simulink model "log_map_tl"  (Simulink 7.5)
settings: Solver=FixedStepDiscrete  StartTime=0.0  StopTime=50.0  FixedStep=0.1  RelTol=1e-3
PreLoadFcn:
  | if exist('tl_preloadfcn','file'), tl_preloadfcn(gcs,101); end
PostLoadFcn:
  | if exist('tl_postloadfcn','file'), tl_postloadfcn(gcs,101); end
InitFcn:
  | if exist('tlds_init','file'), tlds_init(gcs); end
StartFcn:
  | if exist('tlds_start','file'), tlds_start(gcs); end
StopFcn:
  | if exist('tlds_stop','file'), tlds_stop(gcs); end
values from neighbouring files (symbols this model uses):
  alpha = 0.2    [logmap_start.m]
  beta = 0.7    [logmap_start.m]
  lambda = 4.0    (= 4)    [logmap_start.m]
  y1_0 = 0.23421    [logmap_start.m]
  y2_0 = 0.86567    [logmap_start.m]
libraries: tllib x6
PreSaveFcn:
  | if exist('tl_presavefcn','file'), tl_presavefcn(gcs); end
settings Model: DS_PROJECTFILE=log_map_tl.dd  TL_MAIN_DATA={'#advcodeopt',0,'frameopt',{'mexargs',''},'logopt',{'plotinterval',0.1},'date',735991.67651606479}  TL_MODEL_COMMENT=Type in your documentation HERE  TLRevision=101  Creator=alex  LastModifiedBy=alex  BufferReuse=off
settings DataIOCC: LimitDataPoints=off  SaveOutput=off  SaveTime=off
settings OptimizationCC: BlockReduction=off  BooleanDataType=off  OptimizeBlockIOStorage=off  BufferReuse=off  ExpressionFolding=off  LocalBlockOutputs=off  InitFltsAndDblsToZero=on
settings DebuggingCC: SaveWithParameterizedLinksMsg=none  SignalResolutionControl=TryResolveAllWithWarning  SolverPrmCheckMsg=none  MultiTaskDSMMsg=warning  MultiTaskCondExecSysMsg=none
settings HardwareCC: TargetUnknown=on
settings RTWCC: IncludeERTFirstTime=on
settings GRTTargetCC: TargetFcnLib=ansi_tfl_tmw.mat  ModelReferenceCompliant=off  MatFileLogging=off

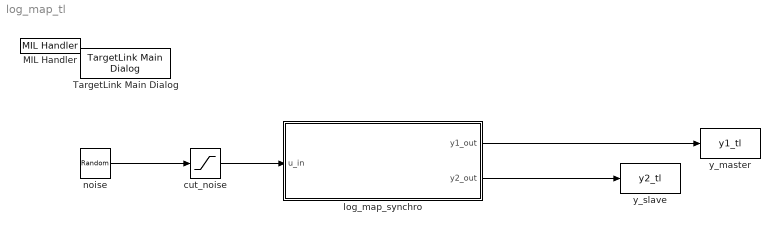
== system log_map_tl ==
  MIL Handler : tllib/MIL Handler  data={'date',735991.67651435186}
  TargetLink Main Dialog : tllib/TargetLink Main Dialog  SystemSampleTime=-1
  cut_noise : Saturate  UpperLimit=1  LowerLimit=0
  log_map_synchro : Subsystem  Tag=TargetLink Simulation Frame
      settings: CopyFcn=if exist('tl_copyfcn','file'), tl_copyfcn(gcbh); end  NameChangeFcn=if exist('tl_framenamechangefcn','file'), tl_framenamechangefcn(gcbh); end
      settings: OpenFcn=|
      | if exist('open_tlsubsystem','file')
      |    open_tlsubsystem(gcbh);
      | else
      |    tlsubsystem = ...
      |       find_system(gcb, ...
      |       'LookUnderMasks','on', ...
      |       'FollowLinks','on', ...
      |       'Tag','MIL Subsystem');
      |    open_system(tlsubsystem);
      | end
      mask Type: TL_SimFrame
      mask Display: disp('TargetLink\nModel-\nin-the-loop\nmode')
  noise : RandomNumber  Mean=0.5  SampleTime=0
  y_master : ToWorkspace  VariableName=y1_tl  SampleTime=-1  SaveFormat=Array
  y_slave : ToWorkspace  VariableName=y2_tl  SampleTime=-1  SaveFormat=Array
  wires:
  noise/1 -> cut_noise/1
  log_map_synchro/1(y1_out) -> y_master/1
  cut_noise/1 -> log_map_synchro/1(u_in)
  log_map_synchro/2(y2_out) -> y_slave/1

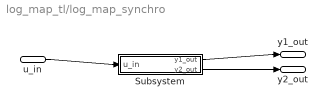
== system log_map_tl/log_map_synchro ==
  u_in : Inport  SampleTime=0.1  OutDataType=sfix(16)  OutScaling=2^0
  Subsystem : Subsystem  Tag=struct('sfcnName','log_map_synchro_sf','subFunction','','srcSubsystem','')
      settings: OpenFcn=warndlg(get_param(gcb,'MaskHelp'),'Serious Warning');
      mask Type: TL_Enable
      mask Help: This subsystem keeps the TargetLink subsystem (subsystem with TargetLink blocks for production code generation), and is needed for the TargetLink simulation frame to work properly. DO NOT DELETE OR MODIFY IT!
  y1_out : Outport  OutDataType=sfix(16)  OutScaling=2^0
  y2_out : Outport  Port=2  OutDataType=sfix(16)  OutScaling=2^0
  wires:
  u_in/1 -> Subsystem/1(u_in)
  Subsystem/1(y1_out) -> y1_out/1
  Subsystem/2(y2_out) -> y2_out/1

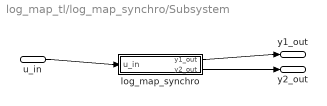
== system log_map_tl/log_map_synchro/Subsystem ==
  u_in : Inport  SampleTime=0.1  OutDataType=sfix(16)  OutScaling=2^0
  log_map_synchro : Subsystem  Tag=MIL Subsystem  Description=b
      settings: CopyFcn=if exist('tl_copyfcn','file'), tl_copyfcn(gcbh); end  NameChangeFcn=if exist('tl_namechangefcn','file'), tl_namechangefcn(gcbh); end  DestroyFcn=if exist('update_tl_main_dlg','file'), update_tl_main_dlg('TL_subs_display'); end
  y1_out : Outport  OutDataType=sfix(16)  OutScaling=2^0
  y2_out : Outport  Port=2  OutDataType=sfix(16)  OutScaling=2^0
  wires:
  u_in/1 -> log_map_synchro/1(u_in)
  log_map_synchro/1(y1_out) -> y1_out/1
  log_map_synchro/2(y2_out) -> y2_out/1

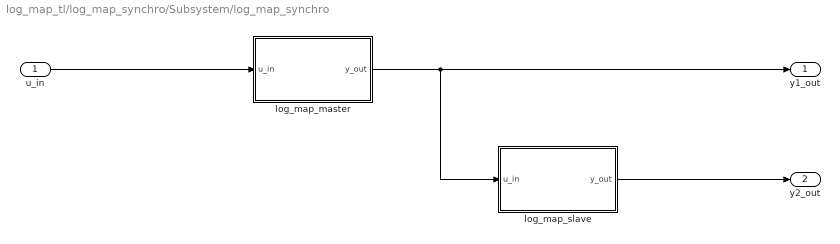
== system log_map_tl/log_map_synchro/Subsystem/log_map_synchro ==
  u_in : Inport  Description=|  PortDimensions=1  SampleTime=0.1  OutDataType=sfix(16)  OutScaling=2^0  mask(TL_Inport){data={'logdata',{'plotchannels',[]},'output',{'max',1,'min',0,'type','UInt16','lsb',2^-15},'date',735991.67651483801}}
      | InPort block of dSPACE TargetLink.
      | 
      | Input signal is read from an external variable and scaled:
      | 
      |         y = lsb * u + offset
      settings: DeleteFcn=if exist('delete_tlblock','file')==2,delete_tlblock(gcbh);end  OpenFcn=if exist('tl_open_blockdlg','file')==2,tl_open_blockdlg(gcbh);else,open_system(gcbh,'parameter');end
      settings: CopyFcn=|
      | if exist('tl_reset_reviewflag','file')==2
      |     tl_reset_reviewflag(gcbh);
      | end
      | if exist('tl_check_ports','file')
      |     tl_check_ports(gcbh);
      | end
      settings: NameChangeFcn=|
      | if exist('rename_tlblock','file')==2,rename_tlblock(gcbh);end
      | if exist('tl_check_ports','file'), tl_check_ports(gcbh); end
      mask Help: eval(['if exist(''tl_online_help'',''file'') == 2, tl_online_help(''Topic'',''TL_Inport''),else, web([''jar:file:///'',matlabroot,''/help/toolbox/simulink/help.jar!/slref/' lower(get_param(gcbh,'Blocktype')) '.html''], ''-helpbrowser''),end'])
      mask Display: plot([0.2 0.35 NaN 0.65 0.8],[0 1 NaN 0 1]);
  log_map_master : Subsystem  TreatAsAtomicUnit=on
  log_map_slave : Subsystem  TreatAsAtomicUnit=on
  y1_out : Outport  Description=|  PortDimensions=1  OutDataType=sfix(16)  OutScaling=2^0  mask(TL_Outport){data={'logdata',{'plotchannels',[]},'output',{'max',1,'min',0,'type','UInt16','lsb',2^-15},'date',735991.67650769674}}
      | OutPort block of dSPACE TargetLink.
      | 
      | Input signal is scaled:
      | 
      |         y = lsb * u + offset
      settings: DeleteFcn=if exist('delete_tlblock','file')==2,delete_tlblock(gcbh);end  OpenFcn=if exist('tl_open_blockdlg','file')==2,tl_open_blockdlg(gcbh);else,open_system(gcbh,'parameter');end
      settings: CopyFcn=|
      | if exist('tl_reset_reviewflag','file')==2
      |     tl_reset_reviewflag(gcbh);
      | end
      | if exist('tl_check_ports','file')
      |     tl_check_ports(gcbh);
      | end
      settings: NameChangeFcn=|
      | if exist('rename_tlblock','file')==2,rename_tlblock(gcbh);end
      | if exist('tl_check_ports','file'), tl_check_ports(gcbh); end
      mask Help: eval(['if exist(''tl_online_help'',''file'') == 2, tl_online_help(''Topic'',''TL_Outport''),else, web([''jar:file:///'',matlabroot,''/help/toolbox/simulink/help.jar!/slref/' lower(get_param(gcbh,'Blocktype')) '.html''], ''-helpbrowser''),end'])
      mask Display: plot([0.2 0.35 NaN 0.65 0.8],[0 1 NaN 0 1]);
  y2_out : Outport  Description=|  Port=2  PortDimensions=1  OutDataType=sfix(16)  OutScaling=2^0  mask(TL_Outport){data={'logdata',{'plotchannels',[]},'output',{'max',1,'min',0,'type','UInt16','lsb',2^-15},'date',735991.67650722223}}
      | OutPort block of dSPACE TargetLink.
      | 
      | Input signal is scaled:
      | 
      |         y = lsb * u + offset
      settings: DeleteFcn=if exist('delete_tlblock','file')==2,delete_tlblock(gcbh);end  OpenFcn=if exist('tl_open_blockdlg','file')==2,tl_open_blockdlg(gcbh);else,open_system(gcbh,'parameter');end
      settings: CopyFcn=|
      | if exist('tl_reset_reviewflag','file')==2
      |     tl_reset_reviewflag(gcbh);
      | end
      | if exist('tl_check_ports','file')
      |     tl_check_ports(gcbh);
      | end
      settings: NameChangeFcn=|
      | if exist('rename_tlblock','file')==2,rename_tlblock(gcbh);end
      | if exist('tl_check_ports','file'), tl_check_ports(gcbh); end
      mask Help: eval(['if exist(''tl_online_help'',''file'') == 2, tl_online_help(''Topic'',''TL_Outport''),else, web([''jar:file:///'',matlabroot,''/help/toolbox/simulink/help.jar!/slref/' lower(get_param(gcbh,'Blocktype')) '.html''], ''-helpbrowser''),end'])
      mask Display: plot([0.2 0.35 NaN 0.65 0.8],[0 1 NaN 0 1]);
  wires:
  log_map_master/1(y_out) -> log_map_slave/1(u_in), y1_out/1
  u_in/1 -> log_map_master/1(u_in)
  log_map_slave/1(y_out) -> y2_out/1

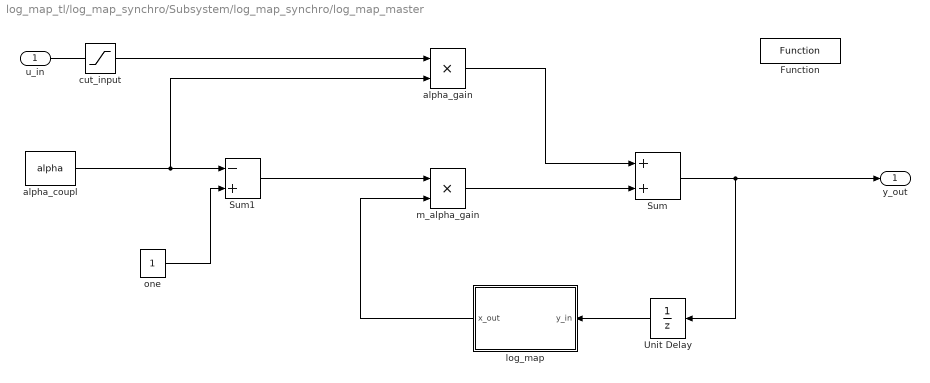
== system log_map_tl/log_map_synchro/Subsystem/log_map_synchro/log_map_master ==
  u_in : Inport  OutDataType=sfix(16)  OutScaling=2^0
  Function : tllib/Function  Description=|  SystemSampleTime=-1  data={'date',735991.6765065972}
      | Function block of dSPACE TargetLink.
      | 
      | Copy this block into a subsystem if you want separate code to be generated for it.
  Sum : Sum  Description=|  OutDataType=sfix(16)  OutScaling=2^-10  mask(TL_Sum){data={'logdata',{'plotchannels',[]},'output',{'max',1,'min',0,'type','UInt16','lsb',2^-15},'date',735991.67651423614}}
      | Sum block of dSPACE TargetLink.
      | 
      | Output signal is equal to the sum of the input signals.
      | The list of signs is specified according to conventions for Simulink Sum blocks.
      settings: CopyFcn=set_param(gcb,'ReferenceBlock',''); set_param(gcb,'Tag','COPIED_DURING_UPGRADE');set_param(gcb,'CopyFcn','');  DeleteFcn=if exist('delete_tlblock','file')==2,delete_tlblock(gcbh);end  NameChangeFcn=if exist('rename_tlblock','file')==2,rename_tlblock(gcbh);end  OpenFcn=if exist('tl_open_blockdlg','file')==2,tl_open_blockdlg(gcbh);else,open_system(gcbh,'parameter');end
      mask Help: eval(['if exist(''tl_online_help'',''file'') == 2, tl_online_help(''Topic'',''TL_Sum''),else, web([''jar:file:///'',matlabroot,''/help/toolbox/simulink/help.jar!/slref/' lower(get_param(gcbh,'Blocktype')) '.html''], ''-helpbrowser''),end'])
      mask Display: plot([-0.05, 1.05, NaN, -0.05, 1.05],[.01, .01, NaN, .99, .99])
  Sum1 : Sum  Description=|  Inputs=-+  OutDataType=sfix(16)  OutScaling=2^-10  mask(TL_Sum){data={'logdata',{'plotchannels',[]},'output',{'max',1,'type','UInt16','lsb',2^-15},'date',735991.67651399306}}
      | Sum block of dSPACE TargetLink.
      | 
      | Output signal is equal to the sum of the input signals.
      | The list of signs is specified according to conventions for Simulink Sum blocks.
      settings: CopyFcn=set_param(gcb,'ReferenceBlock',''); set_param(gcb,'Tag','COPIED_DURING_UPGRADE');set_param(gcb,'CopyFcn','');  DeleteFcn=if exist('delete_tlblock','file')==2,delete_tlblock(gcbh);end  NameChangeFcn=if exist('rename_tlblock','file')==2,rename_tlblock(gcbh);end  OpenFcn=if exist('tl_open_blockdlg','file')==2,tl_open_blockdlg(gcbh);else,open_system(gcbh,'parameter');end
      mask Help: eval(['if exist(''tl_online_help'',''file'') == 2, tl_online_help(''Topic'',''TL_Sum''),else, web([''jar:file:///'',matlabroot,''/help/toolbox/simulink/help.jar!/slref/' lower(get_param(gcbh,'Blocktype')) '.html''], ''-helpbrowser''),end'])
      mask Display: plot([-0.05, 1.05, NaN, -0.05, 1.05],[.01, .01, NaN, .99, .99])
  Unit Delay : UnitDelay  Description=|  X0=y1_0  SampleTime=-1  mask(TL_UnitDelay){data={'logdata',{'plotchannels',[]},'output',{'max',1,'min',0,'type','UInt16','lsb',2^-15},'state',{'max',1,'min',0,'type','UInt16','lsb',2^-15},'date',735991.67651372682}}
      | Unit Delay block of dSPACE TargetLink.
      | 
      | Output signal is equal to the input signal of the last sample step:
      | 
      |         y(k) = u(k-1).
      | 
      | In the 1st sampling step, the output signal is initialized with 'initial condition':
      | 
      |         y(0) = initial condition
      settings: CopyFcn=set_param(gcb,'ReferenceBlock',''); set_param(gcb,'Tag','COPIED_DURING_UPGRADE');set_param(gcb,'CopyFcn','');  DeleteFcn=if exist('delete_tlblock','file')==2,delete_tlblock(gcbh);end  NameChangeFcn=if exist('rename_tlblock','file')==2,rename_tlblock(gcbh);end  OpenFcn=if exist('tl_open_blockdlg','file')==2,tl_open_blockdlg(gcbh);else,open_system(gcbh,'parameter');end
      mask Help: eval(['if exist(''tl_online_help'',''file'') == 2, tl_online_help(''Topic'',''TL_UnitDelay''),else, web([''jar:file:///'',matlabroot,''/help/toolbox/simulink/help.jar!/slref/' lower(get_param(gcbh,'Blocktype')) '.html''], ''-helpbrowser''),end'])
      mask Display: plot([-0.05, 1.05, NaN, -0.05, 1.05],[.01, .01, NaN, .99, .99])
  alpha_coupl : Constant  Description=|  Value=alpha  OutDataType=sfix(16)  OutScaling=2^0  mask(TL_Constant){data={'output',{'max',1,'min',0,'class','CAL','type','UInt16','lsb',2^-15},'date',735991.67651340272}}
      | Constant block of dSPACE TargetLink.
      | 
      | Output signal keeps the given constant value.
      settings: CopyFcn=set_param(gcb,'ReferenceBlock',''); set_param(gcb,'Tag','COPIED_DURING_UPGRADE');set_param(gcb,'CopyFcn','');  DeleteFcn=if exist('delete_tlblock','file')==2,delete_tlblock(gcbh);end  NameChangeFcn=if exist('rename_tlblock','file')==2,rename_tlblock(gcbh);end  OpenFcn=if exist('tl_open_blockdlg','file')==2,tl_open_blockdlg(gcbh);else,open_system(gcbh,'parameter');end
      mask Help: eval(['if exist(''tl_online_help'',''file'') == 2, tl_online_help(''Topic'',''TL_Constant''),else, web([''jar:file:///'',matlabroot,''/help/toolbox/simulink/help.jar!/slref/' lower(get_param(gcbh,'Blocktype')) '.html''], ''-helpbrowser''),end'])
      mask Display: plot([-0.05, 1.05, NaN, -0.05, 1.05],[.01, .01, NaN, .99, .99])
  alpha_gain : Product  Description=|  Inputs=**  OutDataType=sfix(16)  OutScaling=2^0  RndMeth=Zero  mask(TL_Product){data={'logdata',{'plotchannels',[]},'output',{'max',1,'min',0,'type','UInt16','lsb',2^-15},'date',735991.67651315976}}
      | Product block of dSPACE TargetLink.
      | 
      | Output signal is equal to the product of the input signals. The input ports are specified according to conventions for Simulink Product blocks.
      settings: CopyFcn=set_param(gcb,'ReferenceBlock',''); set_param(gcb,'Tag','COPIED_DURING_UPGRADE');set_param(gcb,'CopyFcn','');  DeleteFcn=if exist('delete_tlblock','file')==2,delete_tlblock(gcbh);end  NameChangeFcn=if exist('rename_tlblock','file')==2,rename_tlblock(gcbh);end  OpenFcn=if exist('tl_open_blockdlg','file')==2,tl_open_blockdlg(gcbh);else,open_system(gcbh,'parameter');end
      mask Help: eval(['if exist(''tl_online_help'',''file'') == 2, tl_online_help(''Topic'',''TL_Product''),else, web([''jar:file:///'',matlabroot,''/help/toolbox/simulink/help.jar!/slref/' lower(get_param(gcbh,'Blocktype')) '.html''], ''-helpbrowser''),end'])
      mask Display: plot([-0.05, 1.05, NaN, -0.05, 1.05],[.01, .01, NaN, .99, .99])
  cut_input : Saturate  Description=|  UpperLimit=1  LowerLimit=0  OutDataType=sfix(16)  OutScaling=2^0  mask(TL_Saturate){data={'logdata',{'plotchannels',[]},'output',{'max',1,'min',0,'type','UInt16','lsb',2^-15},'lowerlimit',{'class','GLOBAL','type','UInt16','lsb',2^-15},'upperlimit',{'class','GLOBAL','type','UInt16','lsb',2^-15},'date',735991.676512882}}
      | Saturation block of dSPACE TargetLink.
      | 
      | The Saturation block saturates its input to the given upper and lower limit.
      settings: CopyFcn=set_param(gcb,'ReferenceBlock',''); set_param(gcb,'Tag','COPIED_DURING_UPGRADE');set_param(gcb,'CopyFcn','');  DeleteFcn=if exist('delete_tlblock','file')==2,delete_tlblock(gcbh);end  NameChangeFcn=if exist('rename_tlblock','file')==2,rename_tlblock(gcbh);end  OpenFcn=if exist('tl_open_blockdlg','file')==2,tl_open_blockdlg(gcbh);else,open_system(gcbh,'parameter');end
      mask Help: eval(['if exist(''tl_online_help'',''file'') == 2, tl_online_help(''Topic'',''TL_Saturate''),else, web([''jar:file:///'',matlabroot,''/help/toolbox/simulink/help.jar!/slref/' lower(get_param(gcbh,'Blocktype')) '.html''], ''-helpbrowser''),end'])
      mask Display: plot([-0.05, 1.05, NaN, -0.05, 1.05],[.01, .01, NaN, .99, .99])
  log_map : Subsystem  TreatAsAtomicUnit=on
  m_alpha_gain : Product  Description=|  Inputs=**  OutDataType=sfix(16)  OutScaling=2^0  RndMeth=Zero  mask(TL_Product){data={'logdata',{'plotchannels',[]},'output',{'max',1,'min',0,'type','UInt16','lsb',2^-15},'date',735991.67651142366}}
      | Product block of dSPACE TargetLink.
      | 
      | Output signal is equal to the product of the input signals. The input ports are specified according to conventions for Simulink Product blocks.
      settings: CopyFcn=set_param(gcb,'ReferenceBlock',''); set_param(gcb,'Tag','COPIED_DURING_UPGRADE');set_param(gcb,'CopyFcn','');  DeleteFcn=if exist('delete_tlblock','file')==2,delete_tlblock(gcbh);end  NameChangeFcn=if exist('rename_tlblock','file')==2,rename_tlblock(gcbh);end  OpenFcn=if exist('tl_open_blockdlg','file')==2,tl_open_blockdlg(gcbh);else,open_system(gcbh,'parameter');end
      mask Help: eval(['if exist(''tl_online_help'',''file'') == 2, tl_online_help(''Topic'',''TL_Product''),else, web([''jar:file:///'',matlabroot,''/help/toolbox/simulink/help.jar!/slref/' lower(get_param(gcbh,'Blocktype')) '.html''], ''-helpbrowser''),end'])
      mask Display: plot([-0.05, 1.05, NaN, -0.05, 1.05],[.01, .01, NaN, .99, .99])
  one : Constant  Description=|  OutDataType=sfix(16)  OutScaling=2^0  mask(TL_Constant){data={'output',{'class','CONST','type','UInt16','lsb',2^-15,'tolerance',0.001},'date',735991.67651119211}}
      | Constant block of dSPACE TargetLink.
      | 
      | Output signal keeps the given constant value.
      settings: CopyFcn=set_param(gcb,'ReferenceBlock',''); set_param(gcb,'Tag','COPIED_DURING_UPGRADE');set_param(gcb,'CopyFcn','');  DeleteFcn=if exist('delete_tlblock','file')==2,delete_tlblock(gcbh);end  NameChangeFcn=if exist('rename_tlblock','file')==2,rename_tlblock(gcbh);end  OpenFcn=if exist('tl_open_blockdlg','file')==2,tl_open_blockdlg(gcbh);else,open_system(gcbh,'parameter');end
      mask Help: eval(['if exist(''tl_online_help'',''file'') == 2, tl_online_help(''Topic'',''TL_Constant''),else, web([''jar:file:///'',matlabroot,''/help/toolbox/simulink/help.jar!/slref/' lower(get_param(gcbh,'Blocktype')) '.html''], ''-helpbrowser''),end'])
      mask Display: plot([-0.05, 1.05, NaN, -0.05, 1.05],[.01, .01, NaN, .99, .99])
  y_out : Outport  OutDataType=sfix(16)  OutScaling=2^0
  wires:
  cut_input/1 -> alpha_gain/1
  m_alpha_gain/1 -> Sum/2
  alpha_gain/1 -> Sum/1
  log_map/1(x_out) -> m_alpha_gain/2
  Sum/1 -> y_out/1, Unit Delay/1
  u_in/1 -> cut_input/1
  Unit Delay/1 -> log_map/1(y_in)
  one/1 -> Sum1/2
  Sum1/1 -> m_alpha_gain/1
  alpha_coupl/1 -> Sum1/1, alpha_gain/2

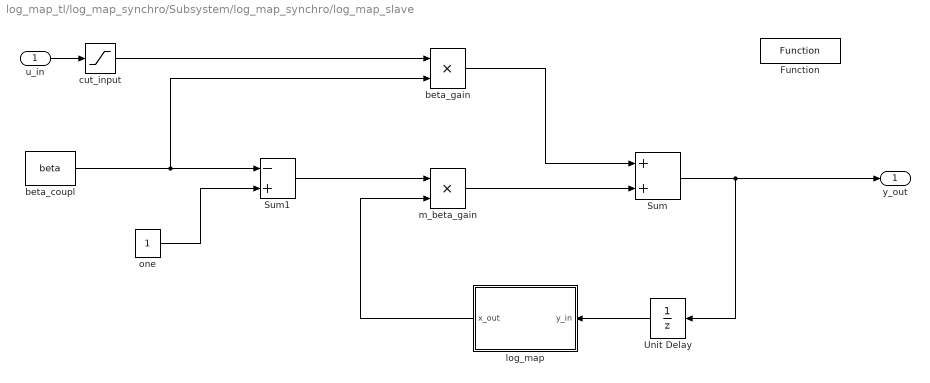
== system log_map_tl/log_map_synchro/Subsystem/log_map_synchro/log_map_slave ==
  u_in : Inport  OutDataType=sfix(16)  OutScaling=2^0
  Function : tllib/Function  Description=|  SystemSampleTime=-1  data={'date',735991.67650611117}
      | Function block of dSPACE TargetLink.
      | 
      | Copy this block into a subsystem if you want separate code to be generated for it.
  Sum : Sum  Description=|  OutDataType=sfix(16)  OutScaling=2^-10  mask(TL_Sum){data={'logdata',{'plotchannels',[]},'output',{'max',1,'min',0,'type','UInt16','lsb',2^-15},'date',735991.67651094904}}
      | Sum block of dSPACE TargetLink.
      | 
      | Output signal is equal to the sum of the input signals.
      | The list of signs is specified according to conventions for Simulink Sum blocks.
      settings: CopyFcn=set_param(gcb,'ReferenceBlock',''); set_param(gcb,'Tag','COPIED_DURING_UPGRADE');set_param(gcb,'CopyFcn','');  DeleteFcn=if exist('delete_tlblock','file')==2,delete_tlblock(gcbh);end  NameChangeFcn=if exist('rename_tlblock','file')==2,rename_tlblock(gcbh);end  OpenFcn=if exist('tl_open_blockdlg','file')==2,tl_open_blockdlg(gcbh);else,open_system(gcbh,'parameter');end
      mask Help: eval(['if exist(''tl_online_help'',''file'') == 2, tl_online_help(''Topic'',''TL_Sum''),else, web([''jar:file:///'',matlabroot,''/help/toolbox/simulink/help.jar!/slref/' lower(get_param(gcbh,'Blocktype')) '.html''], ''-helpbrowser''),end'])
      mask Display: plot([-0.05, 1.05, NaN, -0.05, 1.05],[.01, .01, NaN, .99, .99])
  Sum1 : Sum  Description=|  Inputs=-+  OutDataType=sfix(16)  OutScaling=2^-10  mask(TL_Sum){data={'logdata',{'plotchannels',[]},'output',{'max',1,'type','UInt16','lsb',2^-15},'date',735991.67651068291}}
      | Sum block of dSPACE TargetLink.
      | 
      | Output signal is equal to the sum of the input signals.
      | The list of signs is specified according to conventions for Simulink Sum blocks.
      settings: CopyFcn=set_param(gcb,'ReferenceBlock',''); set_param(gcb,'Tag','COPIED_DURING_UPGRADE');set_param(gcb,'CopyFcn','');  DeleteFcn=if exist('delete_tlblock','file')==2,delete_tlblock(gcbh);end  NameChangeFcn=if exist('rename_tlblock','file')==2,rename_tlblock(gcbh);end  OpenFcn=if exist('tl_open_blockdlg','file')==2,tl_open_blockdlg(gcbh);else,open_system(gcbh,'parameter');end
      mask Help: eval(['if exist(''tl_online_help'',''file'') == 2, tl_online_help(''Topic'',''TL_Sum''),else, web([''jar:file:///'',matlabroot,''/help/toolbox/simulink/help.jar!/slref/' lower(get_param(gcbh,'Blocktype')) '.html''], ''-helpbrowser''),end'])
      mask Display: plot([-0.05, 1.05, NaN, -0.05, 1.05],[.01, .01, NaN, .99, .99])
  Unit Delay : UnitDelay  Description=|  X0=y2_0  SampleTime=-1  mask(TL_UnitDelay){data={'logdata',{'plotchannels',[]},'output',{'max',1,'min',0,'type','UInt16','lsb',2^-15},'state',{'max',1,'min',0,'type','UInt16','lsb',2^-15},'date',735991.67651043984}}
      | Unit Delay block of dSPACE TargetLink.
      | 
      | Output signal is equal to the input signal of the last sample step:
      | 
      |         y(k) = u(k-1).
      | 
      | In the 1st sampling step, the output signal is initialized with 'initial condition':
      | 
      |         y(0) = initial condition
      settings: CopyFcn=set_param(gcb,'ReferenceBlock',''); set_param(gcb,'Tag','COPIED_DURING_UPGRADE');set_param(gcb,'CopyFcn','');  DeleteFcn=if exist('delete_tlblock','file')==2,delete_tlblock(gcbh);end  NameChangeFcn=if exist('rename_tlblock','file')==2,rename_tlblock(gcbh);end  OpenFcn=if exist('tl_open_blockdlg','file')==2,tl_open_blockdlg(gcbh);else,open_system(gcbh,'parameter');end
      mask Help: eval(['if exist(''tl_online_help'',''file'') == 2, tl_online_help(''Topic'',''TL_UnitDelay''),else, web([''jar:file:///'',matlabroot,''/help/toolbox/simulink/help.jar!/slref/' lower(get_param(gcbh,'Blocktype')) '.html''], ''-helpbrowser''),end'])
      mask Display: plot([-0.05, 1.05, NaN, -0.05, 1.05],[.01, .01, NaN, .99, .99])
  beta_coupl : Constant  Description=|  Value=beta  OutDataType=sfix(16)  OutScaling=2^0  mask(TL_Constant){data={'output',{'max',1,'min',0,'class','CAL','type','UInt16','lsb',2^-15},'date',735991.67651011574}}
      | Constant block of dSPACE TargetLink.
      | 
      | Output signal keeps the given constant value.
      settings: CopyFcn=set_param(gcb,'ReferenceBlock',''); set_param(gcb,'Tag','COPIED_DURING_UPGRADE');set_param(gcb,'CopyFcn','');  DeleteFcn=if exist('delete_tlblock','file')==2,delete_tlblock(gcbh);end  NameChangeFcn=if exist('rename_tlblock','file')==2,rename_tlblock(gcbh);end  OpenFcn=if exist('tl_open_blockdlg','file')==2,tl_open_blockdlg(gcbh);else,open_system(gcbh,'parameter');end
      mask Help: eval(['if exist(''tl_online_help'',''file'') == 2, tl_online_help(''Topic'',''TL_Constant''),else, web([''jar:file:///'',matlabroot,''/help/toolbox/simulink/help.jar!/slref/' lower(get_param(gcbh,'Blocktype')) '.html''], ''-helpbrowser''),end'])
      mask Display: plot([-0.05, 1.05, NaN, -0.05, 1.05],[.01, .01, NaN, .99, .99])
  beta_gain : Product  Description=|  Inputs=**  OutDataType=sfix(16)  OutScaling=2^0  RndMeth=Zero  mask(TL_Product){data={'logdata',{'plotchannels',[]},'output',{'max',1,'min',0,'type','UInt16','lsb',2^-15},'date',735991.67650987266}}
      | Product block of dSPACE TargetLink.
      | 
      | Output signal is equal to the product of the input signals. The input ports are specified according to conventions for Simulink Product blocks.
      settings: CopyFcn=set_param(gcb,'ReferenceBlock',''); set_param(gcb,'Tag','COPIED_DURING_UPGRADE');set_param(gcb,'CopyFcn','');  DeleteFcn=if exist('delete_tlblock','file')==2,delete_tlblock(gcbh);end  NameChangeFcn=if exist('rename_tlblock','file')==2,rename_tlblock(gcbh);end  OpenFcn=if exist('tl_open_blockdlg','file')==2,tl_open_blockdlg(gcbh);else,open_system(gcbh,'parameter');end
      mask Help: eval(['if exist(''tl_online_help'',''file'') == 2, tl_online_help(''Topic'',''TL_Product''),else, web([''jar:file:///'',matlabroot,''/help/toolbox/simulink/help.jar!/slref/' lower(get_param(gcbh,'Blocktype')) '.html''], ''-helpbrowser''),end'])
      mask Display: plot([-0.05, 1.05, NaN, -0.05, 1.05],[.01, .01, NaN, .99, .99])
  cut_input : Saturate  Description=|  UpperLimit=1  LowerLimit=0  OutDataType=sfix(16)  OutScaling=2^0  mask(TL_Saturate){data={'logdata',{'plotchannels',[]},'output',{'max',1,'min',0,'type','UInt16','lsb',2^-15},'lowerlimit',{'class','GLOBAL','type','UInt16','lsb',2^-15},'upperlimit',{'class','GLOBAL','type','UInt16','lsb',2^-15},'date',735991.67650961806}}
      | Saturation block of dSPACE TargetLink.
      | 
      | The Saturation block saturates its input to the given upper and lower limit.
      settings: CopyFcn=set_param(gcb,'ReferenceBlock',''); set_param(gcb,'Tag','COPIED_DURING_UPGRADE');set_param(gcb,'CopyFcn','');  DeleteFcn=if exist('delete_tlblock','file')==2,delete_tlblock(gcbh);end  NameChangeFcn=if exist('rename_tlblock','file')==2,rename_tlblock(gcbh);end  OpenFcn=if exist('tl_open_blockdlg','file')==2,tl_open_blockdlg(gcbh);else,open_system(gcbh,'parameter');end
      mask Help: eval(['if exist(''tl_online_help'',''file'') == 2, tl_online_help(''Topic'',''TL_Saturate''),else, web([''jar:file:///'',matlabroot,''/help/toolbox/simulink/help.jar!/slref/' lower(get_param(gcbh,'Blocktype')) '.html''], ''-helpbrowser''),end'])
      mask Display: plot([-0.05, 1.05, NaN, -0.05, 1.05],[.01, .01, NaN, .99, .99])
  log_map : Subsystem  TreatAsAtomicUnit=on
  m_beta_gain : Product  Description=|  Inputs=**  OutDataType=sfix(16)  OutScaling=2^0  RndMeth=Zero  mask(TL_Product){data={'logdata',{'plotchannels',[]},'output',{'max',1,'min',0,'type','UInt16','lsb',2^-15},'date',735991.67650818289}}
      | Product block of dSPACE TargetLink.
      | 
      | Output signal is equal to the product of the input signals. The input ports are specified according to conventions for Simulink Product blocks.
      settings: CopyFcn=set_param(gcb,'ReferenceBlock',''); set_param(gcb,'Tag','COPIED_DURING_UPGRADE');set_param(gcb,'CopyFcn','');  DeleteFcn=if exist('delete_tlblock','file')==2,delete_tlblock(gcbh);end  NameChangeFcn=if exist('rename_tlblock','file')==2,rename_tlblock(gcbh);end  OpenFcn=if exist('tl_open_blockdlg','file')==2,tl_open_blockdlg(gcbh);else,open_system(gcbh,'parameter');end
      mask Help: eval(['if exist(''tl_online_help'',''file'') == 2, tl_online_help(''Topic'',''TL_Product''),else, web([''jar:file:///'',matlabroot,''/help/toolbox/simulink/help.jar!/slref/' lower(get_param(gcbh,'Blocktype')) '.html''], ''-helpbrowser''),end'])
      mask Display: plot([-0.05, 1.05, NaN, -0.05, 1.05],[.01, .01, NaN, .99, .99])
  one : Constant  Description=|  OutDataType=sfix(16)  OutScaling=2^0  mask(TL_Constant){data={'output',{'class','CONST','type','UInt16','lsb',2^-15,'tolerance',0.001},'date',735991.67650795134}}
      | Constant block of dSPACE TargetLink.
      | 
      | Output signal keeps the given constant value.
      settings: CopyFcn=set_param(gcb,'ReferenceBlock',''); set_param(gcb,'Tag','COPIED_DURING_UPGRADE');set_param(gcb,'CopyFcn','');  DeleteFcn=if exist('delete_tlblock','file')==2,delete_tlblock(gcbh);end  NameChangeFcn=if exist('rename_tlblock','file')==2,rename_tlblock(gcbh);end  OpenFcn=if exist('tl_open_blockdlg','file')==2,tl_open_blockdlg(gcbh);else,open_system(gcbh,'parameter');end
      mask Help: eval(['if exist(''tl_online_help'',''file'') == 2, tl_online_help(''Topic'',''TL_Constant''),else, web([''jar:file:///'',matlabroot,''/help/toolbox/simulink/help.jar!/slref/' lower(get_param(gcbh,'Blocktype')) '.html''], ''-helpbrowser''),end'])
      mask Display: plot([-0.05, 1.05, NaN, -0.05, 1.05],[.01, .01, NaN, .99, .99])
  y_out : Outport  OutDataType=sfix(16)  OutScaling=2^0
  wires:
  Unit Delay/1 -> log_map/1(y_in)
  u_in/1 -> cut_input/1
  Sum/1 -> Unit Delay/1, y_out/1
  log_map/1(x_out) -> m_beta_gain/2
  beta_gain/1 -> Sum/1
  m_beta_gain/1 -> Sum/2
  cut_input/1 -> beta_gain/1
  Sum1/1 -> m_beta_gain/1
  beta_coupl/1 -> Sum1/1, beta_gain/2
  one/1 -> Sum1/2

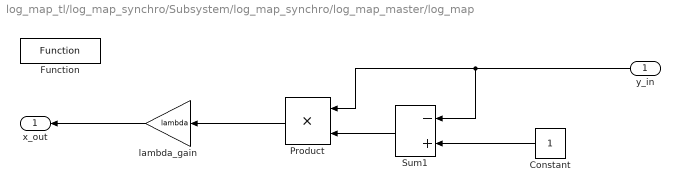
== system log_map_tl/log_map_synchro/Subsystem/log_map_synchro/log_map_master/log_map ==
  y_in : Inport  OutDataType=sfix(16)  OutScaling=2^0
  Constant : Constant  Description=|  OutDataType=sfix(16)  OutScaling=2^0  mask(TL_Constant){data={'output',{'class','CONST','type','UInt16','lsb',2^-15},'date',735991.67651250004}}
      | Constant block of dSPACE TargetLink.
      | 
      | Output signal keeps the given constant value.
      settings: CopyFcn=set_param(gcb,'ReferenceBlock',''); set_param(gcb,'Tag','COPIED_DURING_UPGRADE');set_param(gcb,'CopyFcn','');  DeleteFcn=if exist('delete_tlblock','file')==2,delete_tlblock(gcbh);end  NameChangeFcn=if exist('rename_tlblock','file')==2,rename_tlblock(gcbh);end  OpenFcn=if exist('tl_open_blockdlg','file')==2,tl_open_blockdlg(gcbh);else,open_system(gcbh,'parameter');end
      mask Help: eval(['if exist(''tl_online_help'',''file'') == 2, tl_online_help(''Topic'',''TL_Constant''),else, web([''jar:file:///'',matlabroot,''/help/toolbox/simulink/help.jar!/slref/' lower(get_param(gcbh,'Blocktype')) '.html''], ''-helpbrowser''),end'])
      mask Display: plot([-0.05, 1.05, NaN, -0.05, 1.05],[.01, .01, NaN, .99, .99])
  Function : tllib/Function  Description=|  SystemSampleTime=-1  data={'date',735991.67650635412}
      | Function block of dSPACE TargetLink.
      | 
      | Copy this block into a subsystem if you want separate code to be generated for it.
  Product : Product  Description=|  OutDataType=sfix(16)  OutScaling=2^0  RndMeth=Zero  mask(TL_Product){data={'logdata',{'plotchannels',[]},'output',{'max',1,'min',0,'type','UInt16','lsb',2^-15},'date',735991.67651225696}}
      | Product block of dSPACE TargetLink.
      | 
      | Output signal is equal to the product of the input signals. The input ports are specified according to conventions for Simulink Product blocks.
      settings: CopyFcn=set_param(gcb,'ReferenceBlock',''); set_param(gcb,'Tag','COPIED_DURING_UPGRADE');set_param(gcb,'CopyFcn','');  DeleteFcn=if exist('delete_tlblock','file')==2,delete_tlblock(gcbh);end  NameChangeFcn=if exist('rename_tlblock','file')==2,rename_tlblock(gcbh);end  OpenFcn=if exist('tl_open_blockdlg','file')==2,tl_open_blockdlg(gcbh);else,open_system(gcbh,'parameter');end
      mask Help: eval(['if exist(''tl_online_help'',''file'') == 2, tl_online_help(''Topic'',''TL_Product''),else, web([''jar:file:///'',matlabroot,''/help/toolbox/simulink/help.jar!/slref/' lower(get_param(gcbh,'Blocktype')) '.html''], ''-helpbrowser''),end'])
      mask Display: plot([-0.05, 1.05, NaN, -0.05, 1.05],[.01, .01, NaN, .99, .99])
  Sum1 : Sum  Description=|  Inputs=-+  OutDataType=sfix(16)  OutScaling=2^-10  mask(TL_Sum){data={'logdata',{'plotchannels',[]},'output',{'max',1,'min',0,'type','UInt16','lsb',2^-15},'date',735991.67651202541}}
      | Sum block of dSPACE TargetLink.
      | 
      | Output signal is equal to the sum of the input signals.
      | The list of signs is specified according to conventions for Simulink Sum blocks.
      settings: CopyFcn=set_param(gcb,'ReferenceBlock',''); set_param(gcb,'Tag','COPIED_DURING_UPGRADE');set_param(gcb,'CopyFcn','');  DeleteFcn=if exist('delete_tlblock','file')==2,delete_tlblock(gcbh);end  NameChangeFcn=if exist('rename_tlblock','file')==2,rename_tlblock(gcbh);end  OpenFcn=if exist('tl_open_blockdlg','file')==2,tl_open_blockdlg(gcbh);else,open_system(gcbh,'parameter');end
      mask Help: eval(['if exist(''tl_online_help'',''file'') == 2, tl_online_help(''Topic'',''TL_Sum''),else, web([''jar:file:///'',matlabroot,''/help/toolbox/simulink/help.jar!/slref/' lower(get_param(gcbh,'Blocktype')) '.html''], ''-helpbrowser''),end'])
      mask Display: plot([-0.05, 1.05, NaN, -0.05, 1.05],[.01, .01, NaN, .99, .99])
  lambda_gain : Gain  Description=|  Gain=lambda  ParameterDataType=sfix(16)  ParameterScaling=2^0  OutDataType=sfix(16)  OutScaling=2^0  mask(TL_Gain){data={'logdata',{'plotchannels',[]},'output',{'max',1,'min',0,'type','UInt16','lsb',2^-15},'gain',{'max',4,'min',0,'class','CAL','lsb',2^-12},'date',735991.67651174765}}
      | Gain block of dSPACE TargetLink.
      | 
      | Output signal is equal to the product of the input signal and the gain value:
      |         y = G u
      settings: CopyFcn=set_param(gcb,'ReferenceBlock',''); set_param(gcb,'Tag','COPIED_DURING_UPGRADE');set_param(gcb,'CopyFcn','');  DeleteFcn=if exist('delete_tlblock','file')==2,delete_tlblock(gcbh);end  NameChangeFcn=if exist('rename_tlblock','file')==2,rename_tlblock(gcbh);end  OpenFcn=if exist('tl_open_blockdlg','file')==2,tl_open_blockdlg(gcbh);else,open_system(gcbh,'parameter');end
      mask Help: eval(['if exist(''tl_online_help'',''file'') == 2, tl_online_help(''Topic'',''TL_Gain''),else, web([''jar:file:///'',matlabroot,''/help/toolbox/simulink/help.jar!/slref/' lower(get_param(gcbh,'Blocktype')) '.html''], ''-helpbrowser''),end'])
      mask Display: plot([0, .9, 0],[.05, .5, .95])
  x_out : Outport  OutDataType=sfix(16)  OutScaling=2^0
  wires:
  Constant/1 -> Sum1/2
  Sum1/1 -> Product/2
  y_in/1 -> Sum1/1, Product/1
  Product/1 -> lambda_gain/1
  lambda_gain/1 -> x_out/1

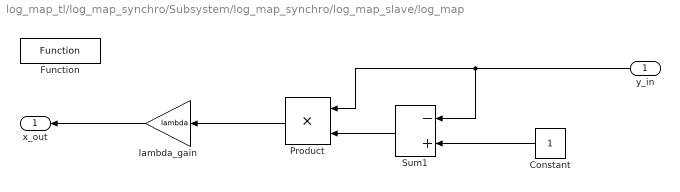
== system log_map_tl/log_map_synchro/Subsystem/log_map_synchro/log_map_slave/log_map ==
  y_in : Inport  OutDataType=sfix(16)  OutScaling=2^0
  Constant : Constant  Description=|  OutDataType=sfix(16)  OutScaling=2^0  mask(TL_Constant){data={'output',{'class','CONST','type','UInt16','lsb',2^-15},'date',735991.67650924763}}
      | Constant block of dSPACE TargetLink.
      | 
      | Output signal keeps the given constant value.
      settings: CopyFcn=set_param(gcb,'ReferenceBlock',''); set_param(gcb,'Tag','COPIED_DURING_UPGRADE');set_param(gcb,'CopyFcn','');  DeleteFcn=if exist('delete_tlblock','file')==2,delete_tlblock(gcbh);end  NameChangeFcn=if exist('rename_tlblock','file')==2,rename_tlblock(gcbh);end  OpenFcn=if exist('tl_open_blockdlg','file')==2,tl_open_blockdlg(gcbh);else,open_system(gcbh,'parameter');end
      mask Help: eval(['if exist(''tl_online_help'',''file'') == 2, tl_online_help(''Topic'',''TL_Constant''),else, web([''jar:file:///'',matlabroot,''/help/toolbox/simulink/help.jar!/slref/' lower(get_param(gcbh,'Blocktype')) '.html''], ''-helpbrowser''),end'])
      mask Display: plot([-0.05, 1.05, NaN, -0.05, 1.05],[.01, .01, NaN, .99, .99])
  Function : tllib/Function  Description=|  SystemSampleTime=-1  data={'date',735991.67650586809}
      | Function block of dSPACE TargetLink.
      | 
      | Copy this block into a subsystem if you want separate code to be generated for it.
  Product : Product  Description=|  OutDataType=sfix(16)  OutScaling=2^0  RndMeth=Zero  mask(TL_Product){data={'logdata',{'plotchannels',[]},'output',{'max',1,'min',0,'type','UInt16','lsb',2^-15},'date',735991.67650901619}}
      | Product block of dSPACE TargetLink.
      | 
      | Output signal is equal to the product of the input signals. The input ports are specified according to conventions for Simulink Product blocks.
      settings: CopyFcn=set_param(gcb,'ReferenceBlock',''); set_param(gcb,'Tag','COPIED_DURING_UPGRADE');set_param(gcb,'CopyFcn','');  DeleteFcn=if exist('delete_tlblock','file')==2,delete_tlblock(gcbh);end  NameChangeFcn=if exist('rename_tlblock','file')==2,rename_tlblock(gcbh);end  OpenFcn=if exist('tl_open_blockdlg','file')==2,tl_open_blockdlg(gcbh);else,open_system(gcbh,'parameter');end
      mask Help: eval(['if exist(''tl_online_help'',''file'') == 2, tl_online_help(''Topic'',''TL_Product''),else, web([''jar:file:///'',matlabroot,''/help/toolbox/simulink/help.jar!/slref/' lower(get_param(gcbh,'Blocktype')) '.html''], ''-helpbrowser''),end'])
      mask Display: plot([-0.05, 1.05, NaN, -0.05, 1.05],[.01, .01, NaN, .99, .99])
  Sum1 : Sum  Description=|  Inputs=-+  OutDataType=sfix(16)  OutScaling=2^-10  mask(TL_Sum){data={'logdata',{'plotchannels',[]},'output',{'max',1,'min',0,'type','UInt16','lsb',2^-15},'date',735991.67650877312}}
      | Sum block of dSPACE TargetLink.
      | 
      | Output signal is equal to the sum of the input signals.
      | The list of signs is specified according to conventions for Simulink Sum blocks.
      settings: CopyFcn=set_param(gcb,'ReferenceBlock',''); set_param(gcb,'Tag','COPIED_DURING_UPGRADE');set_param(gcb,'CopyFcn','');  DeleteFcn=if exist('delete_tlblock','file')==2,delete_tlblock(gcbh);end  NameChangeFcn=if exist('rename_tlblock','file')==2,rename_tlblock(gcbh);end  OpenFcn=if exist('tl_open_blockdlg','file')==2,tl_open_blockdlg(gcbh);else,open_system(gcbh,'parameter');end
      mask Help: eval(['if exist(''tl_online_help'',''file'') == 2, tl_online_help(''Topic'',''TL_Sum''),else, web([''jar:file:///'',matlabroot,''/help/toolbox/simulink/help.jar!/slref/' lower(get_param(gcbh,'Blocktype')) '.html''], ''-helpbrowser''),end'])
      mask Display: plot([-0.05, 1.05, NaN, -0.05, 1.05],[.01, .01, NaN, .99, .99])
  lambda_gain : Gain  Description=|  Gain=lambda  ParameterDataType=sfix(16)  ParameterScaling=2^0  OutDataType=sfix(16)  OutScaling=2^0  mask(TL_Gain){data={'logdata',{'plotchannels',[]},'output',{'max',1,'min',0,'type','UInt16','lsb',2^-15},'gain',{'max',4,'min',0,'class','CAL','lsb',2^-12},'date',735991.67650850699}}
      | Gain block of dSPACE TargetLink.
      | 
      | Output signal is equal to the product of the input signal and the gain value:
      |         y = G u
      settings: CopyFcn=set_param(gcb,'ReferenceBlock',''); set_param(gcb,'Tag','COPIED_DURING_UPGRADE');set_param(gcb,'CopyFcn','');  DeleteFcn=if exist('delete_tlblock','file')==2,delete_tlblock(gcbh);end  NameChangeFcn=if exist('rename_tlblock','file')==2,rename_tlblock(gcbh);end  OpenFcn=if exist('tl_open_blockdlg','file')==2,tl_open_blockdlg(gcbh);else,open_system(gcbh,'parameter');end
      mask Help: eval(['if exist(''tl_online_help'',''file'') == 2, tl_online_help(''Topic'',''TL_Gain''),else, web([''jar:file:///'',matlabroot,''/help/toolbox/simulink/help.jar!/slref/' lower(get_param(gcbh,'Blocktype')) '.html''], ''-helpbrowser''),end'])
      mask Display: plot([0, .9, 0],[.05, .5, .95])
  x_out : Outport  OutDataType=sfix(16)  OutScaling=2^0
  wires:
  lambda_gain/1 -> x_out/1
  Product/1 -> lambda_gain/1
  y_in/1 -> Product/1, Sum1/1
  Sum1/1 -> Product/2
  Constant/1 -> Sum1/2
